simulink model "RRRCartesian"  (R2018b)
settings: Solver=VariableStepAuto  StartTime=0.0  StopTime=8  RelTol=1e-3
settings Model: Creator=Young Wang  LastModifiedBy=Young Wang

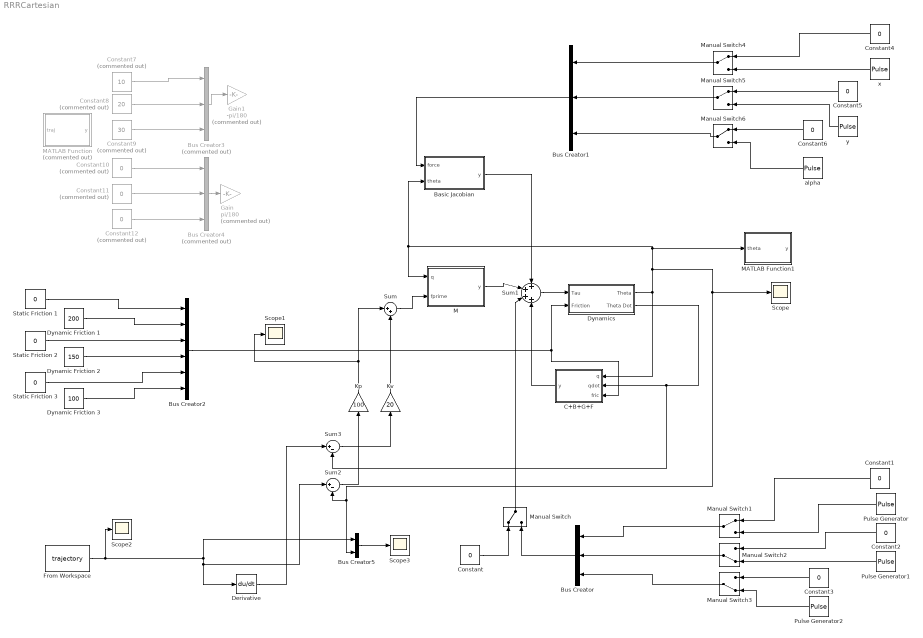
== system RRRCartesian ==
  Basic Jacobian : MATLAB Function  TreatAsAtomicUnit=on
  Bus Creator : BusCreator  Inputs=3
  Bus Creator1 : BusCreator  Inputs=3
  Bus Creator2 : BusCreator  Inputs=6
  Bus Creator3 : BusCreator  Commented=on  Inputs=3
  Bus Creator4 : BusCreator  Commented=on  Inputs=3
  Bus Creator5 : BusCreator  Inputs=2
  C+B+G+F : MATLAB Function  TreatAsAtomicUnit=on
  Constant{,1..6} (7 alike) : Constant  Value=0
  Constant10 : Constant  Commented=on  Value=0
  Constant11 : Constant  Commented=on  Value=0
  Constant12 : Constant  Commented=on  Value=0
  Constant7 : Constant  Commented=on  Value=10
  Constant8 : Constant  Commented=on  Value=20
  Constant9 : Constant  Commented=on  Value=30
  Derivative : Derivative
  Dynamic Friction 1 : Constant  Value=200
  Dynamic Friction 2 : Constant  Value=150
  Dynamic Friction 3 : Constant  Value=100
  Dynamics : Subsystem
  From Workspace : FromWorkspace  VariableName=trajectory  SampleTime=0  OutputAfterFinalValue=Holding final value
  Gain : Gain  Commented=on  Gain=pi/180
  Gain1 : Gain  Commented=on  Gain=-pi/180
  Kp : Gain  Gain=100
  Kv : Gain  Gain=20
  M : MATLAB Function  TreatAsAtomicUnit=on
  MATLAB Function : MATLAB Function  Commented=on  TreatAsAtomicUnit=on
  MATLAB Function1 : MATLAB Function  TreatAsAtomicUnit=on
  Manual Switch{,1,4..6} (5 alike) : ManualSwitch
  Manual Switch2 : ManualSwitch  CurrentSetting=0
  Manual Switch3 : ManualSwitch  CurrentSetting=0
  Pulse Generator : DiscretePulseGenerator  PulseType=Time based  Period=10  PulseWidth=5
  Pulse Generator1 : DiscretePulseGenerator  PulseType=Time based  Period=10  PulseWidth=5
  Pulse Generator2 : DiscretePulseGenerator  PulseType=Time based  Period=10  PulseWidth=5
  Scope{,1..3} (4 alike) : Scope
  Static Friction 1 : Constant  Value=0
  Static Friction 2 : Constant  Value=0
  Static Friction 3 : Constant  Value=0
  Sum : Sum  Inputs=|++
  Sum1 : Sum  Inputs=++++
  Sum2 : Sum  Inputs=|+-
  Sum3 : Sum  Inputs=|+-
  alpha : DiscretePulseGenerator  PulseType=Time based  Period=10  PulseWidth=5
  x : DiscretePulseGenerator  PulseType=Time based  Period=10  PulseWidth=5
  y : DiscretePulseGenerator  PulseType=Time based  Period=10  PulseWidth=5
  wires:
  Sum1/1 -> Dynamics/1(Tau)
  Kp/1 -> Sum/1, Scope1/1
  Kv/1 -> Sum/2
  Dynamics/2(Theta Dot) -> Sum3/2, C+B+G+F/2(qdot)
  Sum/1 -> M/2(fprime)
  Constant/1 -> Manual Switch/1
  Bus Creator/1 -> Manual Switch/2
  Manual Switch1/1 -> Bus Creator/1
  Manual Switch2/1 -> Bus Creator/2
  Manual Switch3/1 -> Bus Creator/3
  Constant1/1 -> Manual Switch1/1
  Constant2/1 -> Manual Switch2/1
  Constant3/1 -> Manual Switch3/1
  Pulse Generator/1 -> Manual Switch1/2
  Pulse Generator1/1 -> Manual Switch2/2
  Pulse Generator2/1 -> Manual Switch3/2
  Manual Switch4/1 -> Bus Creator1/1
  Manual Switch6/1 -> Bus Creator1/3
  alpha/1 -> Manual Switch6/2
  y/1 -> Manual Switch5/2
  Constant5/1 -> Manual Switch5/1
  Constant4/1 -> Manual Switch4/1
  Constant6/1 -> Manual Switch6/1
  x/1 -> Manual Switch4/2
  Manual Switch5/1 -> Bus Creator1/2
  Manual Switch/1 -> Sum1/3
  C+B+G+F/1(y) -> Sum1/4
  M/1(y) -> Sum1/2
  Basic Jacobian/1(y) -> Sum1/1
  Static Friction 3/1 -> Bus Creator2/5
  Dynamic Friction 3/1 -> Bus Creator2/6
  Dynamic Friction 2/1 -> Bus Creator2/4
  Static Friction 2/1 -> Bus Creator2/3
  Dynamic Friction 1/1 -> Bus Creator2/2
  Static Friction 1/1 -> Bus Creator2/1
  Bus Creator2/1 -> C+B+G+F/3(fric), Dynamics/2(Friction)
  Constant7/1 -> Bus Creator3/1
  Constant8/1 -> Bus Creator3/2
  Constant9/1 -> Bus Creator3/3
  Bus Creator1/1 -> Basic Jacobian/1(force)
  Constant12/1 -> Bus Creator4/3
  Constant11/1 -> Bus Creator4/2
  Constant10/1 -> Bus Creator4/1
  Bus Creator4/1 -> Gain/1
  Bus Creator3/1 -> Gain1/1
  Sum2/1 -> Kp/1
  Sum3/1 -> Kv/1
  Dynamics/1(Theta) -> Basic Jacobian/2(theta), M/1(q), MATLAB Function1/1(theta), Scope/1, Bus Creator5/2, Sum2/2, C+B+G+F/1(q)
  From Workspace/1 -> Scope2/1, Bus Creator5/1, Derivative/1, Sum2/1
  Derivative/1 -> Sum3/1
  Bus Creator5/1 -> Scope3/1

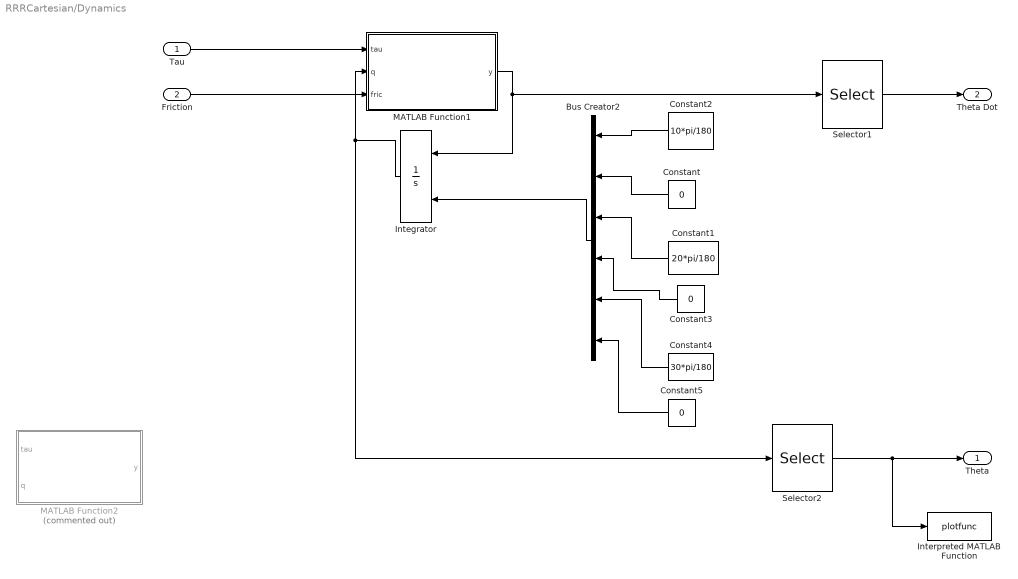
== system RRRCartesian/Dynamics ==
  Tau : Inport
  Friction : Inport  Port=2
  Bus Creator2 : BusCreator  Inputs=6
  Constant : Constant  Value=0
  Constant1 : Constant  Value=20*pi/180
  Constant2 : Constant  Value=10*pi/180
  Constant3 : Constant  Value=0
  Constant4 : Constant  Value=30*pi/180
  Constant5 : Constant  Value=0
  Integrator : Integrator  InitialConditionSource=external
  Interpreted MATLAB Function : MATLABFcn  MATLABFcn=plotfunc  OutputDimensions=0
  MATLAB Function1 : MATLAB Function  TreatAsAtomicUnit=on
  MATLAB Function2 : MATLAB Function  Commented=on  TreatAsAtomicUnit=on
  Selector1 : Selector  InputPortWidth=6  IndexOptions=Index vector (dialog)  Indices=[1 3 5]  OutputSizes=1
  Selector2 : Selector  InputPortWidth=6  IndexOptions=Index vector (dialog)  Indices=[1 3 5]  OutputSizes=1
  Theta : Outport
  Theta Dot : Outport  Port=2
  wires:
  Constant5/1 -> Bus Creator2/6
  Bus Creator2/1 -> Integrator/2
  Constant4/1 -> Bus Creator2/5
  Constant1/1 -> Bus Creator2/3
  Constant3/1 -> Bus Creator2/4
  Integrator/1 -> Selector2/1, MATLAB Function1/2(q)
  Constant/1 -> Bus Creator2/2
  Constant2/1 -> Bus Creator2/1
  MATLAB Function1/1(y) -> Integrator/1, Selector1/1
  Selector1/1 -> Theta Dot/1
  Selector2/1 -> Interpreted MATLAB Function/1, Theta/1
  Tau/1 -> MATLAB Function1/1(tau)
  Friction/1 -> MATLAB Function1/3(fric)

== matlab function RRRCartesian/C+B+G+F ==
  data: q input; qdot input; y output; fric input
function y = fcn(q, qdot,fric)
%parsing for theta
q1 = q(1);
q2 = q(2);
q3 = q(3);

%parsing for theta dot
q1dot = qdot(1);
q2dot = qdot(2);
q3dot = qdot(3);

%parsing for friction
SF1 = fric(1);
SF2 = fric(3);
SF3 = fric(5);
DF1 = fric(2);
DF2 = fric(4);
DF3 = fric(6);

%C matrix
C = zeros(3);
C(1,2) = -40*sin(q2+q3) - 210*sin(q2);
C(1,3) = -40*sin(q2+q3) - 30*sin(q3);
C(2,1) = 40*sin(q2+q3) + 210*sin(q2);
C(2,3) = -30*sin(q3);
C(3,1) = 40*cos(q2+q3) + 30*sin(q3);
C(3,2) = 30*sin(q3);

%B matrix
B = zeros(3);
B(1,1) = -80*sin(q2+q3) - 420*sin(q2);
B(1,2) = -80*sin(q2+q3) -60*sin(q3);
B(1,3) = -80*sin(q2+q3) -60*sin(q3);
B(2,2) = -60*sin(q3);
B(2,3) = -60*sin(q3);
B(3,1) = 60*sin(q3);

%G matrix
G = [0;0;0];
G(1) = (5*9.81*(4*cos(q1 + q2 + q3) + 21*cos(q1 + q2) + 56*cos(q1)))/2;
G(2) = (105*9.81*cos(q1 + q2))/2 + 10*9.81*cos(q1 + q2 + q3);
G(3) = 10*9.81*cos(q1 + q2 + q3);

%F matrix
F = [0;0;0];
F(1)=SF1*sign(q1dot)+DF1*q1dot;
F(2)=SF2*sign(q2dot)+DF2*q2dot;
F(3)=SF3*sign(q3dot)+DF3*q3dot;

%C+B+G+F
V=C*[q1dot;q2dot;q3dot].^2+B*[q1dot*q2dot;q1dot*q3dot;q2dot*q3dot];
y = V+G+F;
end

== matlab function RRRCartesian/M ==
  data: q input; y output; fprime input
function y = fcn(q, fprime)
%parsing for thetas
q1 = q(1);
q2 = q(2);
q3 = q(3);

M = zeros(3);
M(1,1) = 80*cos(q2+q3) + 420*cos(q2) + 60*cos(q3) + (12291/20);
M(1,2) = 40*cos(q2+q3) + 210*cos(q2) + 60*cos(q3) + (2681/20);
M(1,3) = 40*cos(q2+q3) + 30*cos(q3) + (101/10);
M(2,1) = 40*cos(q2+q3) + 210*cos(q2) + 60*cos(q3) + (2681/20);
M(2,2) = 60*cos(q3) + (2681/20);
M(2,3) = 30*cos(q3) + (101/10);
M(3,1) = 40*cos(q2+q3) + 30*cos(q3) + (101/10);
M(3,2) = 30*cos(q3) + (101/10);
M(3,3) = 101/10;
y = M*fprime;
end

== matlab function RRRCartesian/Basic Jacobian ==
  data: force input; y output; theta input
function y = jacobian(force, theta)
%parse theta
q1 = theta(1);
q2 = theta(2);
q3 = theta(3);

%basic jacobian 
J = zeros(3);
J(1,1) = -2*sin(q1+q2+q3) - 3*sin(q1+q2) - 4*sin(q1);
J(1,2) = -2*sin(q1+q2+q3) - 3*sin(q1+q2);
J(1,3) = -2*sin(q1+q2+q3);
J(2,1) = 2*sin(q1+q2+q3) + 3*sin(q1+q2) + 4*sin(q1);
J(2,2) = 2*sin(q1+q2+q3) + 3*sin(q1+q2);
J(2,3) = 2*sin(q1+q2+q3);
J(3,1) = 1;
J(3,2) = 1;
J(3,3) = 1;
y =(J')*force;
end

== matlab function RRRCartesian/Dynamics/MATLAB Function1 ==
  data: tau input; y output; q input; fric input
function y = Dynamics(tau,q,fric)
%parsing q
q1=q(1);
q1dot=q(2);
q2=q(3);
q2dot=q(4);
q3=q(5);
q3dot=q(6);

%Friction Static and Dynamic
SF1 = fric(1);
SF2 = fric(3);
SF3 = fric(5);
DF1 = fric(2);
DF2 = fric(4);
DF3 = fric(6);
%Mass matrix
M = zeros(3);
M(1,1) = 80*cos(q2+q3) + 420*cos(q2) + 60*cos(q3) + (12291/20);
M(1,2) = 40*cos(q2+q3) + 210*cos(q2) + 60*cos(q3) + (2681/20);
M(1,3) = 40*cos(q2+q3) + 30*cos(q3) + (101/10);
M(2,1) = 40*cos(q2+q3) + 210*cos(q2) + 60*cos(q3) + (2681/20);
M(2,2) = 60*cos(q3) + (2681/20);
M(2,3) = 30*cos(q3) + (101/10);
M(3,1) = 40*cos(q2+q3) + 30*cos(q3) + (101/10);
M(3,2) = 30*cos(q3) + (101/10);
M(3,3) = 101/10;

%C matrix
C = zeros(3);
C(1,2) = -40*sin(q2+q3) - 210*sin(q2);
C(1,3) = -40*sin(q2+q3) - 30*sin(q3);
C(2,1) = 40*sin(q2+q3) + 210*sin(q2);
C(2,3) = -30*sin(q3);
C(3,1) = 40*cos(q2+q3) + 30*sin(q3);
C(3,2) = 30*sin(q3);

%B matrix
B = zeros(3);
B(1,1) = -80*sin(q2+q3) - 420*sin(q2);
B(1,2) = -80*sin(q2+q3) -60*sin(q3);
B(1,3) = -80*sin(q2+q3) -60*sin(q3);
B(2,2) = -60*sin(q3);
B(2,3) = -60*sin(q3);
B(3,1) = 60*sin(q3);

%G matrix
G = [0;0;0];
G(1) = (5*9.81*(4*cos(q1 + q2 + q3) + 21*cos(q1 + q2) + 56*cos(q1)))/2;
G(2) = (105*9.81*cos(q1 + q2))/2 + 10*9.81*cos(q1 + q2 + q3);
G(3) = 10*9.81*cos(q1 + q2 + q3);

%F matrix
F = [0;0;0];
F(1)=SF1*sign(q1dot)+DF1*q1dot;
F(2)=SF2*sign(q2dot)+DF2*q2dot;
F(3)=SF3*sign(q3dot)+DF3*q3dot;

%Solving for acceleration
V=C*[q1dot;q2dot;q3dot].^2+B*[q1dot*q2dot;q1dot*q3dot;q2dot*q3dot];
qdd=pinv(M)*(tau-V-G-F);
y=[q1dot;qdd(1);q2dot;qdd(2);q3dot;qdd(3)];
end

== matlab function RRRCartesian/Dynamics/MATLAB Function2 ==
  data: tau input; q input; y output
function y=RRR(tau,q)
% %syms l1 l2 l3 m1 m2 m3
% syms q1 q2 q3
% syms tau
% 
% syms q1dot q2dot q3dot 
q1=q(1);
q1dot=q(2);
q2=q(3);
q2dot=q(4);
q3=q(5);
q3dot=q(6);
V=zeros(3,1);

s1=sin(q1);
c1=cos(q1);
s2=sin(q2);
c2=cos(q2);
s3=sin(q3);
c3=cos(q3);

s12=sin(q1+q2);
c12=cos(q1+q2);

s23=sin(q2+q3);
c23=cos(q2+q3);

s123=sin(q1+q2+q3);
c123=cos(q1+q2+q3);

SF1=200;
DF1=0;

SF2=150;
DF2=0;

SF3=100;
DF3=0;

% syms g real
% syms a real
% m=[a]; %note m is 3 by 3 by 3
% b=[a]; %note b is 3 by 3 by 3
% C=[a]; %note C is 3 by 3
% B=[a]; %note b is 3 by 3

%syms b111 b122 133 real
%syms b211 b222 b233 real
%syms b311 b322 b333 real

l1 = 4;
l2 = 3;
l3 = 2;
m1 = 20;
m2 = 15;
m3 = 10;
ic1 = 0.5;
ic2 = 0.2;
ic3 = 0.1;
%%
%transformation matrices
trans01 = [cos(q1) -sin(q1) 0 0; sin(q1) cos(q1) 0 0; 0 0 1 0; 0 0 0 1];
trans12 = [cos(q2) -sin(q2) 0 l1; sin(q2) cos(q2) 0 0; 0 0 1 0; 0 0 0 1];
trans23 = [cos(q3) -sin(q3) 0 l2; sin(q3) cos(q3) 0 0; 0 0 1 0; 0 0 0 1];
trans3E = [1 0 0 l3; 0 1 0 0; 0 0 1 0; 0 0 0 1];

%pcn point
pc1 = [l1/2; 0; 0; 1];
pc2 = [l2/2; 0; 0; 1];
pc3 = [l3/2; 0; 0; 1];
pcE = [0; 0; 0; 1];

%transposed pcn point
transPc1 = trans01*pc1;
transPc2 = trans01*trans12*pc2;
transPc3 = trans01*trans12*trans23*pc3;
transPcE = trans01*trans12*trans23*trans3E*pcE;

transPc1 = transPc1';
transPc2 = transPc2';
transPc3 = transPc3';

%jacobian 
% jv1 = jacobian(transPc1(1:3), [q1 q2 q3]);
% jv2 = jacobian(transPc2(1:3), [q1 q2 q3]);
% jv3 = jacobian(transPc3(1:3), [q1 q2 q3]);

% jv1_1= diff(transPc1(1:3), q1);
% jv1_2= diff(transPc1(1:3), q2);
% jv1_3 = diff(transPc1(1:3), q3);


jv1=zeros(3,3);
jv1(1,1)=-2*s1;
jv1(2,1)=2*c1;

% jv1=[jv1_1(1) jv1_2(1) jv1_3(1); jv1_1(2) jv1_2(2) jv1_3(2); jv1_1(3) jv1_2(3) jv1_3(3)]


jv2=[-(3*s12)/2-4*s1 -(3*s12)/2 0;
     3*c12/2+4*c1 3*c12/2  0;
     0 0 0];

 jv3=[-s123-3*s12-4*s1 -s123-3*s12 -s123;
      s123+3*c12+4*c1 c123+3*c12 c123;
      0 0 0];
% jv2_1= diff(transPc2(1:3), q1);
% jv2_2= diff(transPc2(1:3), q2);
% jv2_3 = diff(transPc2(1:3), q3);
% jv2=[jv2_1(1) jv2_2(1) jv2_3(1); jv2_1(2) jv2_2(2) jv2_3(2); jv2_1(3) jv2_2(3) jv2_3(3)]

% jv3_1= diff(transPc3(1:3), q1);
% jv3_2= diff(transPc3(1:3), q2);
% jv3_3 = diff(transPc3(1:3), q3);
% jv3=[jv3_1(1) jv3_2(1) jv3_3(1); jv3_1(2) jv3_2(2) jv3_3(2); jv3_1(3) jv3_2(3) jv3_3(3)]
% jv1 = simplify(jv1);
% jv2 = simplify(jv2);
% jv3 = simplify(jv3);

jw1 = [0 0 0; 0 0 0; 1 0 0];
jw2 = [0 0 0; 0 0 0; 1 1 0];
jw3 = [0 0 0; 0 0 0; 1 1 1];

%inertial matrix
Ic1 = [0 0 0; 0 0 0; 0 0 ic1];
Ic2 = [0 0 0; 0 0 0; 0 0 ic2];
Ic3 = [0 0 0; 0 0 0; 0 0 ic3];

%mass matrix
mv1 = jv1'*jv1*m1;
mv2 = jv2'*jv2*m2;
mv3 = jv3'*jv3*m3;
mw1 = jw1'*Ic1*jw1;
mw2 = jw2'*Ic2*jw2;
mw3 = jw3'*Ic3*jw3;

mtotal = mv1+mv2+mv3+mw1+mw2+mw3;


% m11 = mtotal(1,1);
% m12 = mtotal(1,2);
% m13 = mtotal(1,3);
% m21 = mtotal(2,1);
% m22 = mtotal(2,2);
% m23 = mtotal(2,3);
% m31 = mtotal(3,1);
% m32 = mtotal(3,2);
% m33 = mtotal(3,3);

%%
g=9.81;
GMatrix=-(jv1'*[0;-m1*g;0]+(jv2'*[0;-m2*g;0])+(jv3'*[0;-m3*g;0]));


%%


%1st row b(ijk)=1/2*(mijk+mikj-mjki)
% m=zeros(3,3,3);


% for i=1:3
%     for j=1:3
%     m(i,j,1)=diff(mtotal(i,j),q1);  %calculate m111 m211 m311
%     m(i,j,2)=diff(mtotal(i,j),q2);  %calculate m122 m222 m322
%     m(i,j,3)=diff(mtotal(i,j),q3);  %calculate m133 m233 m333
%     end 
% end 

%%
% b=zeros(3,3,3);
% for i=1:3
%     for j=1:3
%         for k=1:3
%             b(i,j,k)=1/2*(m(i,j,k)+m(i,k,j)-m(j,k,i));
%         end 
%     end 
% end 
% C=zeros(3,3);
% for i=1:3
%     for j=1:3
%       C(i,j)=b(i,j,j);
%     end 
% end 


% B=zeros(3,3);
% for i=1:3
%     for j=1:2
%       B(i,j)=2*b(i,1,j+1);
%     end 
% end 
% 
% B(1,3)=2*b(1,2,3);
% B(2,3)=2*b(2,2,3);
% B(3,3)=2*b(3,2,3);

J1F=SF1*sign(q1dot)+DF1*q1dot;
J2F=SF2*sign(q2dot)+DF2*q2dot;
J3F=SF3*sign(q3dot)+DF3*q3dot;
F=[J1F;J2F;J3F];

C=[0        -40*s23-210*s2      -40*s23-30*s3;
    40*s23+210*s2   0           -30*s3;
    40*s23+30*s3    30*s3              0];
B=[-80*s23-420*s2 -80*s23-60*s3 -80*s23-60*s3;
    0               -60*s3          -60*s3;
    0                   0               60*s3];

V=C*[q1dot;q2dot;q3dot].^2+B*[q1dot*q2dot;q1dot*q3dot;q2dot*q3dot];
qdd=pinv(mtotal)*(tau-V-GMatrix-F);


y=[q1dot;qdd(1);q2dot;qdd(2);q3dot;qdd(3)];
end

== matlab function RRRCartesian/MATLAB Function ==
  data: y output; traj input
function y = fcn(traj)
%parsing traj
time = traj(:,1);
q1s = traj(:,2);
q2s = traj(:,3);
q3s = traj(:,4);

for i = 1:801
        q1=q1s(i);
        q2=q2s(i);
        q3=q3s(i);
        vect = [q1; q2; q3];
        y = vect;
end

y = [0; 0; 0];
end

== matlab function RRRCartesian/MATLAB Function1 ==
  data: theta input; y output
function y = fcn(theta)
q1 = theta(1);
q2 = theta(2);
q3 = theta(3);
T0_E = [cos(q1 + q2 + q3)  -sin(q1 + q2 + q3)  0  2*cos(q1+q2+q3)+3*cos(q1+q2) 
y = ;
